simulink model "stateflowrpiv2"  (R2024a)
settings: Solver=FixedStepAuto  StartTime=0.0  StopTime=10.0  RelTol=1e-3  EnableMultiTasking=on
values from neighbouring files (symbols this model uses):
  apps1AdcMax = 30000.0    [rfr25rpi_datadict.sldd]
  apps1AdcMin = 5000.0    [rfr25rpi_datadict.sldd]
  apps2AdcMax = 2000.0    [rfr25rpi_datadict.sldd]
  apps2AdcMin = 1000.0    [rfr25rpi_datadict.sldd]
  cmdTorqueMax = 0.0    [rfr25rpi_datadict.sldd]
  cmdTorqueMin = 5.0    [rfr25rpi_datadict.sldd]
  FDR = 3.77    [rfr25rpi_datadict.sldd]
  MotorRPMtoSpeed = 0.02346    [rfr25rpi_datadict.sldd]
undefined symbols (not defined in the file or in its folder): A0, A2, A3, ended, GND, Single
libraries: raspberrypiBasiclib x9, canmsglib x7, simulink x4, raspberrypiCommlib x3
settings Model: DataDictionary=rfr25rpi_datadict.sldd  ExtModeTrigDuration=2  Creator=user  LastModifiedBy=user
settings SolverCC: PositivePriorityOrder=on
settings OptimizationCC: EnhancedBackFolding=on  PassReuseOutputArgsAs=Individual arguments  ZeroExternalMemoryAtStartup=off  ZeroInternalMemoryAtStartup=off  MaxStackSize=64  OptimizeBlockOrder=speed  DifferentSizesBufferReuse=on  OptimizationCustomize=off  EfficientTunableParamExpr=on
settings DebuggingCC: ParameterTunabilityLossMsg=error
settings HardwareCC: ProdBitPerPointer=32  ProdBitPerSizeT=32  ProdBitPerPtrDiffT=32  ProdLargestAtomicInteger=Long  ProdLargestAtomicFloat=Double  ProdWordSize=32  ProdLongLongMode=on  ProdHWDeviceType=ARM Compatible->ARM Cortex
settings RTWCC: Description=Embedded Coder  SystemTargetFile=ert.tlc  HardwareBoard=Raspberry Pi  TLCOptions="-aInlineSetEventsForThisBaseRateFcn=TLC_FALSE -aSuppressMultiTaskScheduler=TLC_FALSE  -aRateBasedStepFcn=0"  TemplateMakefile=ert_default_tmf  Toolchain=GNU GCC Embedded Linux  BuildConfiguration=Faster Runs
settings CodeAppCC: ForceParamTrailComments=on  IgnoreCustomStorageClasses=off  OperatorAnnotations=on  SimulinkDataObjDesc=on  SFDataObjDesc=on  InsertBlockDesc=on
settings ERTTargetCC: SupportVariableSizeSignals=on

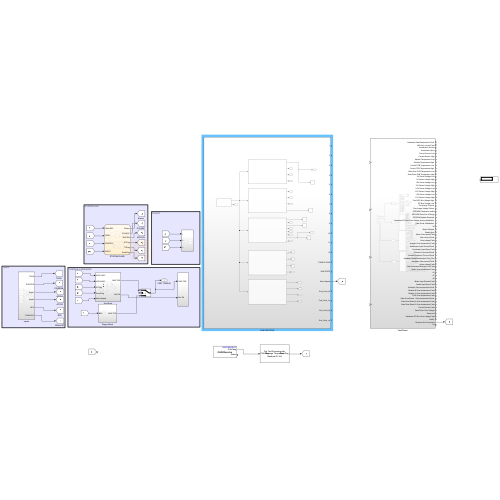
[thumbnail: Simulink's stored preview of the top-level diagram]
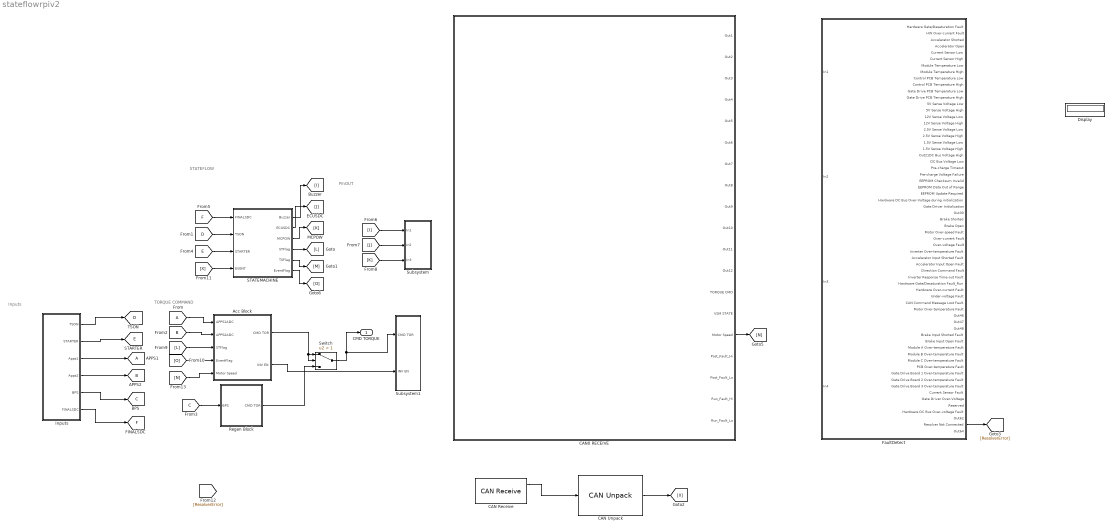
== system stateflowrpiv2 ==
  note: STATEFLOW
  note: TORQUE COMMAND
  note: Inputs
  note: PinOUT
  APPS1 : Goto  TagVisibility=global
  Acc Block : Subsystem
  CAN Receive : raspberrypiCommlib/CAN Receive  DeviceID=can1  SetupCAN=off  TypeofCAN=Real  OutputDataType=CAN Msg  IdentifierType=Standard (11-bit identifier)  MessageId=100  MsgLength=8  SampleTime=-1  OutputError=off  OutputRemote=off  SimulateUsing=Code generation
  CAN Unpack : canmsglib/CAN Unpack  CANdbFile=E:\EE2025\TestTorquemap.dbc  MsgList=TorqueMap  MsgName=TorqueMap  MsgIDType=Standard (11-bit identifier)  MsgIdentifier=244  MsgLength=1  SignalInfo={'EventFlag','0','8','LE','unsigned','Standard','0','1','0','0','255'}  IDPort=off  TimestampPort=off  ErrorPort=off  RemotePort=off  LengthPort=off  StatusPort=off  ApplyMinMax=off
      settings: LibrarySourceBlock=canlib/CAN Unpack  DataFormat=CANdb specified signals
  CAN0 RECEIVE : Subsystem
  Display : Display
  FaultDetect : Subsystem
  From : From  TagVisibility=global
  Inputs : Subsystem
  Regen Block : Subsystem
  STATEMACHINE : Stateflow chart  TreatAsAtomicUnit=on
      settings: PortSchema="{\"entries\":[{\"content\":{\"sides\":[{\"content\":{\"connectorIds\":[\"In1\",\"In2\",\"In3\",\"In4\"]},\"type\":\"ConnectorPlacement.EquallySpacedRectSide\",\"uuid\":\"0f8b280b-7cb1-472e-a5ac-e36a5d7bcf1b\"},{\"content\":{\"connectorIds\":[\"Out1\",\"Out5\",\"Out3\",\"Out4\",\"Out2\",\"Out6\"],\"side\":\"RIGHT\"},\"type\":\"ConnectorPlacement.EquallySpacedRectSide\",\"uuid\":\"0b1c52b6-a8da-4f2c-8787-2a587349ccd1\"},{\"content\":{\"side\":\"TOP\"},\"type\":\"ConnectorPlacement.EquallySpacedRectSide\",\"uuid\":\"6fa40707-83f4-478b-9f22-811819b1809f\"}]},\"type\":\"ConnectorPlacement.EquallySpacedConnector\",\"uuid\":\"b2952a38-a560-4999-b9e3-ff289dd499fe\"}],\"packageUris\":[\"http://schema.mathworks.com/mf0/Connector/R2020b\"],\"version\":\"1.0\"}"
  Subsystem : Subsystem
  Subsystem1 : Subsystem
  Switch : Switch  Criteria=u2 > Threshold  Threshold=1  SaturateOnIntegerOverflow=off  InputSameDT=off
  CMD TORQUE : Outport
  tag scope: B=global, C=global, D=global, E=global, F=global
  wires:
  [L] -> Acc Block/3(STFlag)
  [E] -> STATEMACHINE/3(STARTER)
  Regen Block/1(CMD TOR) -> Switch/3
  STATEMACHINE/2(TSFlag) -> [M]
  Acc Block/2(INV EN) -> Subsystem1/2(INV EN)
  Inputs/2(STARTER) -> [E]
  STATEMACHINE/5(ECUSDC) -> [J]
  STATEMACHINE/1(Buzzer) -> [I]
  Inputs/6(FINALSDC) -> [F]
  [J] -> Subsystem/2(In2)
  [D] -> STATEMACHINE/2(TSON)
  Inputs/3(Apps1) -> APPS1/1
  Inputs/1(TSON) -> [D]
  [C] -> Regen Block/1(BPS)
  STATEMACHINE/3(MCPOW) -> [K]
  [I] -> Subsystem/1(In1)
  Inputs/4(Apps2) -> [B]
  [F] -> STATEMACHINE/1(FINALSDC)
  [B] -> Acc Block/2(APPS2ADC)
  Inputs/5(BPS) -> [C]
  [K] -> Subsystem/3(In3)
  Acc Block/1(CMD TOR) -> Switch/2, Switch/1
  STATEMACHINE/4(STFlag) -> [L]
  From/1 -> Acc Block/1(APPS1ADC)
  Switch/1 -> CMD TORQUE/1, Subsystem1/1(CMD TOR)
  [N] -> Acc Block/5(Motor Speed)
  STATEMACHINE/6(EventFlag) -> [O]
  [O] -> Acc Block/4(EventFlag)
  CAN0 RECEIVE/15(Motor Speed) -> [N]
  CAN Receive/1 -> CAN Unpack/1
  CAN Unpack/1 -> [X]
  [X] -> STATEMACHINE/4(EVENT)
  FaultDetect/63(Resolver Not Connected) -> [ResolverError]

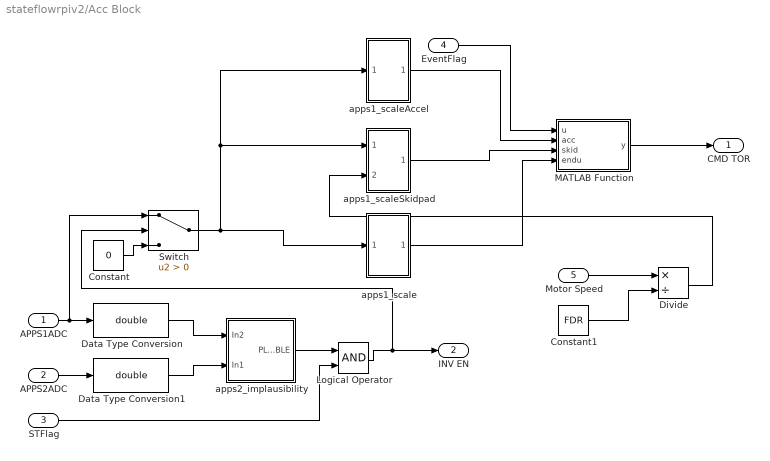
== system stateflowrpiv2/Acc Block ==
  APPS1ADC : Inport
  APPS2ADC : Inport  Port=2
  STFlag : Inport  Port=3
  EventFlag : Inport  Port=4
  Motor Speed : Inport  Port=5
  Constant : Constant  Value=0
  Constant1 : Constant  Value=FDR
  Data Type Conversion : DataTypeConversion  OutDataTypeStr=double  SaturateOnIntegerOverflow=off  RndMeth=Floor
  Data Type Conversion1 : DataTypeConversion  OutDataTypeStr=double  SaturateOnIntegerOverflow=off  RndMeth=Floor
  Divide : Product  Inputs=*/
  Logical Operator : Logic  AllPortsSameDT=off  OutDataTypeStr=boolean
  MATLAB Function : MATLAB Function  TreatAsAtomicUnit=on
  Switch : Switch  Criteria=u2 > Threshold  SaturateOnIntegerOverflow=off  InputSameDT=off
  apps1_scale : Subsystem
  apps1_scaleAccel : Subsystem
  apps1_scaleSkidpad : Subsystem
  apps2_implausibility : Subsystem
  CMD TOR : Outport
  INV EN : Outport  Port=2
  wires:
  APPS1ADC/1 -> Switch/1, Data Type Conversion/1
  APPS2ADC/1 -> Data Type Conversion1/1
  Data Type Conversion1/1 -> apps2_implausibility/2(In1)
  Data Type Conversion/1 -> apps2_implausibility/1(In2)
  apps2_implausibility/1(PLAUSIBLE) -> Logical Operator/1
  Constant/1 -> Switch/3
  STFlag/1 -> Logical Operator/2
  Logical Operator/1 -> Switch/2, INV EN/1
  Motor Speed/1 -> Divide/1
  Constant1/1 -> Divide/2
  Divide/1 -> apps1_scaleSkidpad/2(In2)
  Switch/1 -> apps1_scale/1(In1), apps1_scaleSkidpad/1(In1), apps1_scaleAccel/1(In1)
  EventFlag/1 -> MATLAB Function/1(u)
  apps1_scaleAccel/1(acc) -> MATLAB Function/2(acc)
  apps1_scaleSkidpad/1(skid) -> MATLAB Function/3(skid)
  apps1_scale/1(endu) -> MATLAB Function/4(endu)
  MATLAB Function/1(y) -> CMD TOR/1

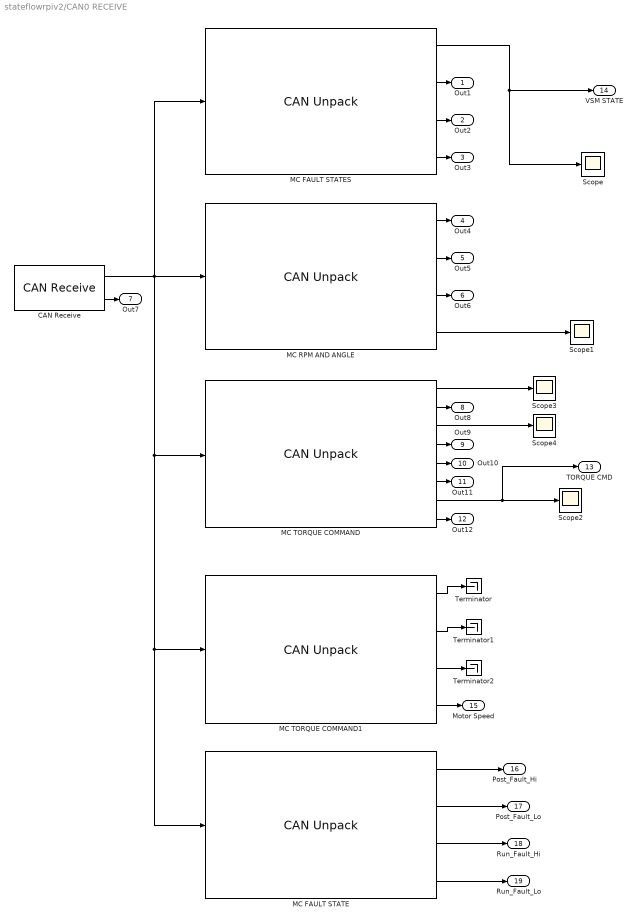
== system stateflowrpiv2/CAN0 RECEIVE ==
  CAN Receive : raspberrypiCommlib/CAN Receive  DeviceID=can0  SetupCAN=on  TypeofCAN=Real  OutputDataType=CAN Msg  IdentifierType=Standard (11-bit identifier)  MessageId=100  MsgLength=8  SampleTime=-1  OutputError=off  OutputRemote=off  SimulateUsing=Code generation
  MC FAULT STATE : canmsglib/CAN Unpack  CANdbFile=C:\Users\user\Desktop\rfr25can0.dbc  MsgList=M171_Fault_Codes  MsgName=M171_Fault_Codes  MsgIDType=Standard (11-bit identifier)  MsgIdentifier=171  MsgLength=8  SignalInfo={'INV_Post_Fault_Hi','16','16','LE','unsigned','Standard','0','1','0','0','65535';'INV_Post_Fault_Lo','0','16','LE','unsigned','Standard','0','1','0','0','65535';'INV_Run_Fault_Hi','48','16','LE','unsigned','Standard','0','1','0','0','65535';'INV_Run_Fault_Lo','32','16','LE','unsigned','Standard','0','1','0','0','65535'}  IDPort=off  TimestampPort=off  ErrorPort=off  RemotePort=off  LengthPort=off  StatusPort=off  ApplyMinMax=off
      settings: LibrarySourceBlock=canlib/CAN Unpack  DataFormat=CANdb specified signals
  MC FAULT STATES : canmsglib/CAN Unpack  CANdbFile=C:\Users\1724a\OneDrive\Desktop\rfr\rfr25can0.dbc  MsgList=(none)  MsgName=M171_Fault_Codes  MsgIDType=Standard (11-bit identifier)  MsgIdentifier=171  MsgLength=8  SignalInfo={'INV_Post_Fault_Hi','16','16','LE','unsigned','Standard','0','1','0','0','65535';'INV_Post_Fault_Lo','0','16','LE','unsigned','Standard','0','1','0','0','65535';'INV_Run_Fault_Hi','48','16','LE','unsigned','Standard','0','1','0','0','65535';'INV_Run_Fault_Lo','32','16','LE','unsigned','Standard','0','1','0','0','65535'}  IDPort=off  TimestampPort=off  ErrorPort=off  RemotePort=off  LengthPort=off  StatusPort=off  ApplyMinMax=off
      settings: LibrarySourceBlock=canlib/CAN Unpack  DataFormat=CANdb specified signals
  MC RPM AND ANGLE : canmsglib/CAN Unpack  CANdbFile=C:\Users\1724a\OneDrive\Desktop\rfr\rfr25can0.dbc  MsgList=(none)  MsgName=M165_Motor_Position_Info  MsgIDType=Standard (11-bit identifier)  MsgIdentifier=165  MsgLength=8  SignalInfo={'INV_Delta_Resolver_Filtered','48','16','LE','signed','Standard','0','0.1','0','-3276.8','3276.7';'INV_Electrical_Output_Frequency','32','16','LE','signed','Standard','0','0.1','0','-3276.8','3276.7';'INV_Motor_Angle_Electrical','0','16','LE','unsigned','Standard','0','0.1','0','0','6553.5';'INV_Motor_Speed','16','16','LE','signed','Standard','0','1','0','-32768','32767'}  IDPort=off  TimestampPort=off  ErrorPort=off  RemotePort=off  LengthPort=off  StatusPort=off  ApplyMinMax=off
      settings: LibrarySourceBlock=canlib/CAN Unpack  DataFormat=CANdb specified signals
  MC TORQUE COMMAND : canmsglib/CAN Unpack  CANdbFile=C:\Users\1724a\OneDrive\Desktop\rfr\rfr25can0.dbc  MsgList=(none)  MsgName=M192_Command_Message  MsgIDType=Standard (11-bit identifier)  MsgIdentifier=192  MsgLength=8  SignalInfo={'VCU_INV_Direction_Command','32','1','LE','unsigned','Standard','0','1','0','0','1';'VCU_INV_Inverter_Discharge','41','1','LE','unsigned','Standard','0','1','0','0','1';'VCU_INV_Inverter_Enable','40','1','LE','unsigned','Standard','0','1','0','0','1';'VCU_INV_RollingCounter','44','4','LE','unsigned','Standard','0','1','0','0','15';'VCU_INV_Speed_Command','16','16','LE','signed','Standard','0','1','0','-32768','32767';'VCU_INV_Speed_Mode_Enable','42','1','LE','unsigned','Standard','0','1','0','0','1';'VCU_INV_Torque_Command','0','16','LE','signed','Standard','0','0.1','0','-3276.8','3276.7';'VCU_INV_Torque_Limit_Command','48','16','LE','signed','Standard','0','0.1','0','-3276.8','3276.7'}  IDPort=off  TimestampPort=off  ErrorPort=off  RemotePort=off  LengthPort=off  StatusPort=off  ApplyMinMax=off
      settings: LibrarySourceBlock=canlib/CAN Unpack  DataFormat=CANdb specified signals
  MC TORQUE COMMAND1 : canmsglib/CAN Unpack  CANdbFile=C:\Users\user\Desktop\rfr25can0.dbc  MsgList=M165_Motor_Position_Info  MsgName=M165_Motor_Position_Info  MsgIDType=Standard (11-bit identifier)  MsgIdentifier=165  MsgLength=8  SignalInfo={'INV_Delta_Resolver_Filtered','48','16','LE','signed','Standard','0','0.1','0','-3276.8','3276.7';'INV_Electrical_Output_Frequency','32','16','LE','signed','Standard','0','0.1','0','-3276.8','3276.7';'INV_Motor_Angle_Electrical','0','16','LE','unsigned','Standard','0','0.1','0','0','6553.5';'INV_Motor_Speed','16','16','LE','signed','Standard','0','1','0','-32768','32767'}  IDPort=off  TimestampPort=off  ErrorPort=off  RemotePort=off  LengthPort=off  StatusPort=off  ApplyMinMax=off
      settings: LibrarySourceBlock=canlib/CAN Unpack  DataFormat=CANdb specified signals
  Scope{,1..4} (5 alike) : Scope
  Terminator : Terminator
  Terminator1 : Terminator
  Terminator2 : Terminator
  Out1 : Outport
  Out2 : Outport  Port=2
  Out3 : Outport  Port=3
  Out4 : Outport  Port=4
  Out5 : Outport  Port=5
  Out6 : Outport  Port=6
  Out7 : Outport  Port=7
  Out8 : Outport  Port=8
  Out9 : Outport  Port=9
  Out10 : Outport  Port=10
  Out11 : Outport  Port=11
  Out12 : Outport  Port=12
  TORQUE CMD : Outport  Port=13
  VSM STATE : Outport  Port=14
  Motor Speed : Outport  Port=15
  Post_Fault_Hi : Outport  Port=16
  Post_Fault_Lo : Outport  Port=17
  Run_Fault_Hi : Outport  Port=18
  Run_Fault_Lo : Outport  Port=19
  wires:
  MC TORQUE COMMAND/3 -> Scope4/1
  CAN Receive/1 -> MC TORQUE COMMAND1/1, MC FAULT STATE/1, MC TORQUE COMMAND/1, MC FAULT STATES/1, MC RPM AND ANGLE/1
  MC TORQUE COMMAND/8 -> Out12/1
  MC TORQUE COMMAND/4 -> Out9/1
  MC RPM AND ANGLE/2 -> Out5/1
  MC TORQUE COMMAND/1 -> Scope3/1
  MC RPM AND ANGLE/1 -> Out4/1
  MC FAULT STATES/1 -> VSM STATE/1, Scope/1
  MC TORQUE COMMAND/6 -> Out11/1
  MC RPM AND ANGLE/4 -> Scope1/1
  MC FAULT STATES/3 -> Out2/1
  CAN Receive/2 -> Out7/1
  MC FAULT STATES/2 -> Out1/1
  MC TORQUE COMMAND/2 -> Out8/1
  MC FAULT STATES/4 -> Out3/1
  MC TORQUE COMMAND/5 -> Out10/1
  MC RPM AND ANGLE/3 -> Out6/1
  MC TORQUE COMMAND/7 -> TORQUE CMD/1, Scope2/1
  MC TORQUE COMMAND1/4 -> Motor Speed/1
  MC TORQUE COMMAND1/1 -> Terminator/1
  MC TORQUE COMMAND1/2 -> Terminator1/1
  MC TORQUE COMMAND1/3 -> Terminator2/1
  MC FAULT STATE/2 -> Post_Fault_Lo/1
  MC FAULT STATE/3 -> Run_Fault_Hi/1
  MC FAULT STATE/4 -> Run_Fault_Lo/1
  MC FAULT STATE/1 -> Post_Fault_Hi/1

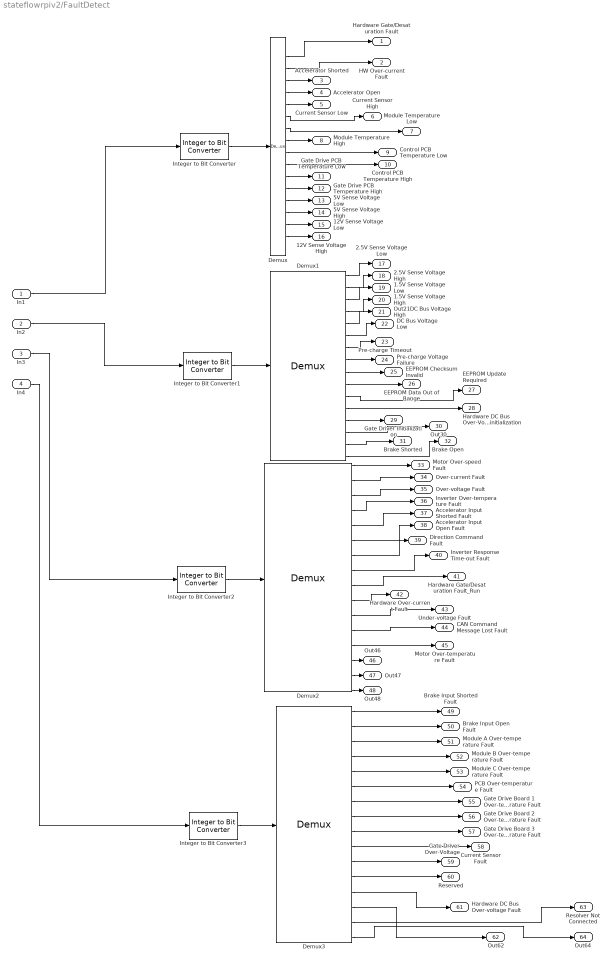
== system stateflowrpiv2/FaultDetect ==
  In1 : Inport
  In2 : Inport  Port=2
  In3 : Inport  Port=3
  In4 : Inport  Port=4
  Demux{,1..3} (4 alike) : Demux  Outputs=16
  Integer to Bit Converter{,1..3} (4 alike) : simulink/Logic and Bit Operations/Integer to Bit Converter  nbits=16  signedInputValues=Unsigned  bitOrder=MSB first  outDtype=Inherit via internal rule
  "Hardware Gate/Desaturation Fault " : Outport
  HW Over-current Fault : Outport  Port=2
  Accelerator Shorted : Outport  Port=3
  Accelerator Open : Outport  Port=4
  Current Sensor Low : Outport  Port=5
  Current Sensor High : Outport  Port=6
  Module Temperature Low : Outport  Port=7
  "Module Temperature High " : Outport  Port=8
  "Control PCB Temperature Low " : Outport  Port=9
  "Control PCB Temperature High " : Outport  Port=10
  Gate Drive PCB Temperature Low : Outport  Port=11
  Gate Drive PCB Temperature High : Outport  Port=12
  5V Sense Voltage Low : Outport  Port=13
  5V Sense Voltage High : Outport  Port=14
  12V Sense Voltage Low : Outport  Port=15
  12V Sense Voltage High : Outport  Port=16
  2.5V Sense Voltage Low : Outport  Port=17
  2.5V Sense Voltage High : Outport  Port=18
  1.5V Sense Voltage Low : Outport  Port=19
  1.5V Sense Voltage High : Outport  Port=20
  "Out21DC Bus Voltage High " : Outport  Port=21
  "DC Bus Voltage Low " : Outport  Port=22
  "Pre-charge Timeout " : Outport  Port=23
  "Pre-charge Voltage Failure " : Outport  Port=24
  EEPROM Checksum Invalid : Outport  Port=25
  EEPROM Data Out of Range : Outport  Port=26
  "EEPROM Update Required " : Outport  Port=27
  "Hardware DC Bus Over-Voltage during initialization " : Outport  Port=28
  "Gate Driver Initialization " : Outport  Port=29
  Out30 : Outport  Port=30
  "Brake Shorted " : Outport  Port=31
  Brake Open : Outport  Port=32
  Motor Over-speed Fault : Outport  Port=33
  "Over-current Fault " : Outport  Port=34
  Over-voltage Fault : Outport  Port=35
  Inverter Over-temperature Fault : Outport  Port=36
  "Accelerator Input Shorted Fault " : Outport  Port=37
  Accelerator Input Open Fault : Outport  Port=38
  "Direction Command Fault " : Outport  Port=39
  "Inverter Response Time-out Fault " : Outport  Port=40
  Hardware Gate/Desaturation Fault_Run : Outport  Port=41
  "Hardware Over-current Fault " : Outport  Port=42
  Under-voltage Fault : Outport  Port=43
  CAN Command Message Lost Fault : Outport  Port=44
  Motor Over-temperature Fault : Outport  Port=45
  Out46 : Outport  Port=46
  Out47 : Outport  Port=47
  Out48 : Outport  Port=48
  Brake Input Shorted Fault : Outport  Port=49
  Brake Input Open Fault : Outport  Port=50
  "Module A Over-temperature Fault " : Outport  Port=51
  Module B Over-temperature Fault : Outport  Port=52
  Module C Over-temperature Fault : Outport  Port=53
  PCB Over-temperature Fault : Outport  Port=54
  "Gate Drive Board 1 Over-temperature Fault " : Outport  Port=55
  Gate Drive Board 2 Over-temperature Fault : Outport  Port=56
  Gate Drive Board 3 Over-temperature Fault : Outport  Port=57
  Current Sensor Fault : Outport  Port=58
  Gate Driver Over-Voltage : Outport  Port=59
  Reserved : Outport  Port=60
  Hardware DC Bus Over-voltage Fault : Outport  Port=61
  "Out62 " : Outport  Port=62
  Resolver Not Connected : Outport  Port=63
  Out64 : Outport  Port=64
  wires:
  Demux2/7 -> "Direction Command Fault "/1
  Demux3/9 -> Gate Drive Board 3 Over-temperature Fault/1
  Integer to Bit Converter1/1 -> Demux1/1
  Demux/4 -> Accelerator Open/1
  Demux/2 -> HW Over-current Fault/1
  Demux1/14 -> Out30/1
  Demux/13 -> 5V Sense Voltage Low/1
  Demux/9 -> "Control PCB Temperature Low "/1
  Demux2/1 -> Motor Over-speed Fault/1
  Demux3/2 -> Brake Input Open Fault/1
  Demux/3 -> Accelerator Shorted/1
  Integer to Bit Converter/1 -> Demux/1
  Demux3/13 -> Hardware DC Bus Over-voltage Fault/1
  Demux1/15 -> "Brake Shorted "/1
  Demux1/9 -> EEPROM Checksum Invalid/1
  Demux1/12 -> "Hardware DC Bus Over-Voltage during initialization "/1
  Demux/5 -> Current Sensor Low/1
  Demux2/10 -> "Hardware Over-current Fault "/1
  Demux/15 -> 12V Sense Voltage Low/1
  Demux/6 -> Current Sensor High/1
  Integer to Bit Converter2/1 -> Demux2/1
  Demux2/13 -> Motor Over-temperature Fault/1
  Integer to Bit Converter3/1 -> Demux3/1
  Demux/16 -> 12V Sense Voltage High/1
  In1/1 -> Integer to Bit Converter/1
  Demux/14 -> 5V Sense Voltage High/1
  Demux1/3 -> 1.5V Sense Voltage Low/1
  Demux3/7 -> "Gate Drive Board 1 Over-temperature Fault "/1
  Demux1/1 -> 2.5V Sense Voltage Low/1
  Demux3/8 -> Gate Drive Board 2 Over-temperature Fault/1
  Demux2/5 -> "Accelerator Input Shorted Fault "/1
  Demux1/6 -> "DC Bus Voltage Low "/1
  Demux2/8 -> "Inverter Response Time-out Fault "/1
  Demux3/5 -> Module C Over-temperature Fault/1
  Demux/11 -> Gate Drive PCB Temperature Low/1
  Demux/8 -> "Module Temperature High "/1
  Demux3/12 -> Reserved/1
  Demux3/1 -> Brake Input Shorted Fault/1
  Demux1/16 -> Brake Open/1
  Demux1/13 -> "Gate Driver Initialization "/1
  Demux/7 -> Module Temperature Low/1
  Demux/1 -> "Hardware Gate/Desaturation Fault "/1
  Demux2/6 -> Accelerator Input Open Fault/1
  Demux2/2 -> "Over-current Fault "/1
  Demux3/4 -> Module B Over-temperature Fault/1
  Demux1/5 -> "Out21DC Bus Voltage High "/1
  Demux2/14 -> Out46/1
  Demux3/3 -> "Module A Over-temperature Fault "/1
  Demux/12 -> Gate Drive PCB Temperature High/1
  Demux1/10 -> EEPROM Data Out of Range/1
  Demux1/8 -> "Pre-charge Voltage Failure "/1
  Demux2/3 -> Over-voltage Fault/1
  Demux2/4 -> Inverter Over-temperature Fault/1
  Demux2/9 -> Hardware Gate/Desaturation Fault_Run/1
  Demux3/6 -> PCB Over-temperature Fault/1
  In2/1 -> Integer to Bit Converter1/1
  Demux3/14 -> "Out62 "/1
  Demux1/11 -> "EEPROM Update Required "/1
  Demux1/7 -> "Pre-charge Timeout "/1
  Demux1/4 -> 1.5V Sense Voltage High/1
  In4/1 -> Integer to Bit Converter3/1
  Demux3/16 -> Out64/1
  Demux3/11 -> Gate Driver Over-Voltage/1
  Demux3/10 -> Current Sensor Fault/1
  Demux/10 -> "Control PCB Temperature High "/1
  Demux2/15 -> Out47/1
  Demux1/2 -> 2.5V Sense Voltage High/1
  Demux2/11 -> Under-voltage Fault/1
  Demux2/12 -> CAN Command Message Lost Fault/1
  Demux2/16 -> Out48/1
  Demux3/15 -> Resolver Not Connected/1
  In3/1 -> Integer to Bit Converter2/1

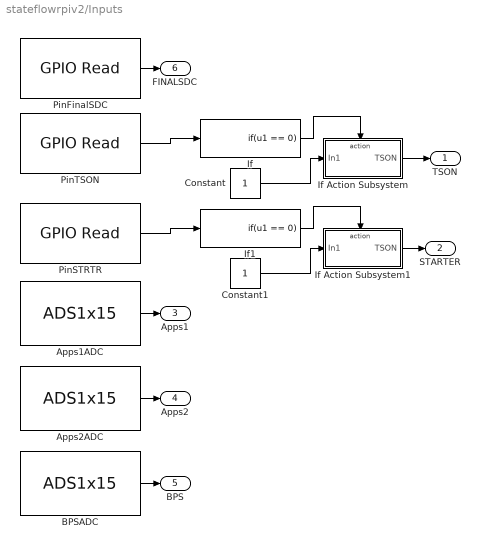
== system stateflowrpiv2/Inputs ==
  Apps1ADC : raspberrypiBasiclib/ADS1x15  ADCChip=ADS1115  I2CAddress=0x48  ConversionMode=Single-shot  InputConfiguration=A2 - GND (Single-ended)  GainConfigurationDifferential=+/- 2.048 V  GainConfigurationSingleEnded=1.024 V  DataRateConfigurationADS1015=1600SPS  DataRateConfigurationADS1115=860SPS  SampleTime=0.1  EnableComparatorMode=off  ComparatorMode=Traditional with hysterisis  ComparatorPolarityConfiguration=Active low  ComparatorLatchingConfiguration=Non-latching  ComparatorQueueConfiguration=Assert after 1 conversion  ComparatorLowThresholdADS1015=0  ComparatorLowThresholdADS1115=0  ComparatorHighThresholdADS1015=0  ComparatorHighThresholdADS1115=0
  Apps2ADC : raspberrypiBasiclib/ADS1x15  ADCChip=ADS1115  I2CAddress=0x48  ConversionMode=Single-shot  InputConfiguration=A3 - GND (Single-ended)  GainConfigurationDifferential=+/- 2.048 V  GainConfigurationSingleEnded=1.024 V  DataRateConfigurationADS1015=1600SPS  DataRateConfigurationADS1115=860SPS  SampleTime=0.1  EnableComparatorMode=off  ComparatorMode=Traditional with hysterisis  ComparatorPolarityConfiguration=Active low  ComparatorLatchingConfiguration=Non-latching  ComparatorQueueConfiguration=Assert after 1 conversion  ComparatorLowThresholdADS1015=0  ComparatorLowThresholdADS1115=0  ComparatorHighThresholdADS1015=0  ComparatorHighThresholdADS1115=0
  BPSADC : raspberrypiBasiclib/ADS1x15  ADCChip=ADS1115  I2CAddress=0x48  ConversionMode=Single-shot  InputConfiguration=A0 - GND (Single-ended)  GainConfigurationDifferential=+/- 2.048 V  GainConfigurationSingleEnded=1.024 V  DataRateConfigurationADS1015=1600SPS  DataRateConfigurationADS1115=860SPS  SampleTime=0.1  EnableComparatorMode=off  ComparatorMode=Traditional with hysterisis  ComparatorPolarityConfiguration=Active low  ComparatorLatchingConfiguration=Non-latching  ComparatorQueueConfiguration=Assert after 1 conversion  ComparatorLowThresholdADS1015=0  ComparatorLowThresholdADS1115=0  ComparatorHighThresholdADS1015=0  ComparatorHighThresholdADS1115=0
  Constant : Constant
  Constant1 : Constant
  If : If  IfExpression=u1 == 0  ShowElse=off
  If Action Subsystem : Subsystem  TreatAsAtomicUnit=on
  If Action Subsystem1 : Subsystem  TreatAsAtomicUnit=on
  If1 : If  IfExpression=u1 == 0  ShowElse=off
  PinFinalSDC : raspberrypiBasiclib/GPIO Read  board=Pi Zero 2 W  gpio=5  internalResistor=Off  sampleTime=0.1  direction=Input  blockPlatform=Raspberry Pi
  PinSTRTR : raspberrypiBasiclib/GPIO Read  board=Pi Zero 2 W  gpio=12  internalResistor=Off  sampleTime=0.1  direction=Input  blockPlatform=Raspberry Pi
  PinTSON : raspberrypiBasiclib/GPIO Read  board=Pi Zero 2 W  gpio=13  internalResistor=Off  sampleTime=0.1  direction=Input  blockPlatform=Raspberry Pi
  TSON : Outport
  STARTER : Outport  Port=2
  Apps1 : Outport  Port=3
  Apps2 : Outport  Port=4
  BPS : Outport  Port=5
  FINALSDC : Outport  Port=6
  wires:
  Apps2ADC/1 -> Apps2/1
  Apps1ADC/1 -> Apps1/1
  BPSADC/1 -> BPS/1
  PinFinalSDC/1 -> FINALSDC/1
  PinTSON/1 -> If/1
  If/1 -> If Action Subsystem/Action
  Constant/1 -> If Action Subsystem/1(In1)
  If Action Subsystem/1(TSON) -> TSON/1
  PinSTRTR/1 -> If1/1
  If Action Subsystem1/1(TSON) -> STARTER/1
  Constant1/1 -> If Action Subsystem1/1(In1)
  If1/1 -> If Action Subsystem1/Action

== system stateflowrpiv2/Regen Block ==
  BPS : Inport
  Data Type Conversion : DataTypeConversion  OutDataTypeStr=double  SaturateOnIntegerOverflow=off  RndMeth=Floor
  Scope : Scope
  Scope1 : Scope
  apps_scale : Subsystem
  CMD TOR : Outport
  wires:
  Data Type Conversion/1 -> apps_scale/1(In1), Scope/1
  apps_scale/1(Out1) -> CMD TOR/1, Scope1/1
  BPS/1 -> Data Type Conversion/1

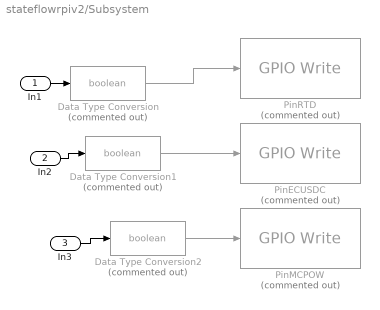
== system stateflowrpiv2/Subsystem ==
  In1 : Inport
  In2 : Inport  Port=2
  In3 : Inport  Port=3
  Data Type Conversion : DataTypeConversion  Commented=on  OutDataTypeStr=boolean  SaturateOnIntegerOverflow=off  RndMeth=Floor
  Data Type Conversion1 : DataTypeConversion  Commented=on  OutDataTypeStr=boolean  SaturateOnIntegerOverflow=off  RndMeth=Floor
  Data Type Conversion2 : DataTypeConversion  Commented=on  OutDataTypeStr=boolean  SaturateOnIntegerOverflow=off  RndMeth=Floor
  PinECUSDC : raspberrypiBasiclib/GPIO Write  Commented=on  board=Pi Zero 2 W  gpio=17  direction=Output  blockPlatform=Raspberry Pi
  PinMCPOW : raspberrypiBasiclib/GPIO Write  Commented=on  board=Pi Zero 2 W  gpio=6  direction=Output  blockPlatform=Raspberry Pi
  PinRTD : raspberrypiBasiclib/GPIO Write  Commented=on  board=Pi Zero 2 W  gpio=25  direction=Output  blockPlatform=Raspberry Pi
  wires:
  In1/1 -> Data Type Conversion/1
  Data Type Conversion/1 -> PinRTD/1
  Data Type Conversion1/1 -> PinECUSDC/1
  In2/1 -> Data Type Conversion1/1
  Data Type Conversion2/1 -> PinMCPOW/1
  In3/1 -> Data Type Conversion2/1

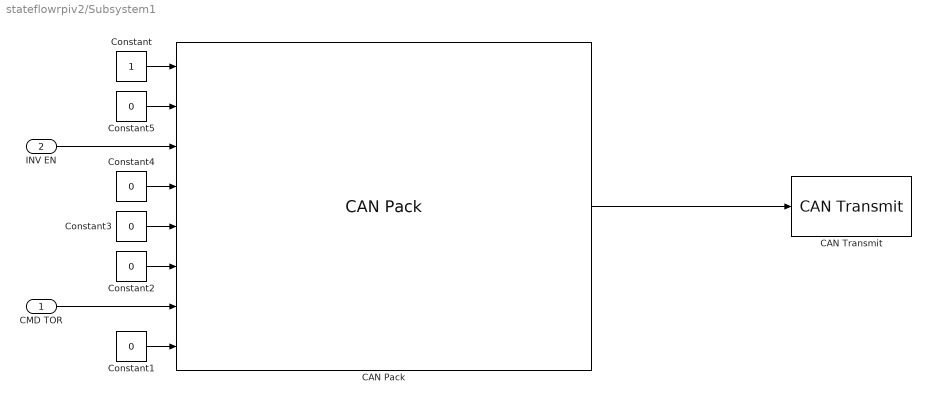
== system stateflowrpiv2/Subsystem1 ==
  CMD TOR : Inport
  INV EN : Inport  Port=2
  CAN Pack : canmsglib/CAN Pack  CANdbFile=C:\Users\user\Desktop\rfr25can0.dbc  MsgList=(none)  MsgName=M192_Command_Message  MsgIDType=Standard (11-bit identifier)  MsgIdentifier=192  MsgLength=8  Remote=off  ApplyMinMax=off  BusOutput=on  SignalInfo={'VCU_INV_Direction_Command','32','1','LE','unsigned','Standard','0','1','0','0','1';'VCU_INV_Inverter_Discharge','41','1','LE','unsigned','Standard','0','1','0','0','1';'VCU_INV_Inverter_Enable','40','1','LE','unsigned','Standard','0','1','0','0','1';'VCU_INV_RollingCounter','44','4','LE','unsigned','Standard','0','1','0','0','15';'VCU_INV_Speed_Command','16','16','LE','signed','Standard','0','1','0','-32768','32767';'VCU_INV_Speed_Mode_Enable','42','1','LE','unsigned','Standard','0','1','0','0','1';'VCU_INV_Torque_Command','0','16','LE','signed','Standard','0','0.1','0','-3276.8','3276.7';'VCU_INV_Torque_Limit_Command','48','16','LE','signed','Standard','0','0.1','0','-3276.8','3276.7'}
      settings: LibrarySourceBlock=canlib/CAN Pack  DataFormat=CANdb specified signals
  CAN Transmit : raspberrypiCommlib/CAN Transmit  DeviceID=can0  SetupCAN=on  TypeofCAN=Real  InputDataType=CAN Msg  BlockingMode_=on  BlockTimeout_=100  OutputStatus=off  IdentifierType=Standard (11-bit identifier)  MessageId=192  MsgLength=8  RemoteFrame=off  SimulateUsing=Code generation
  Constant : Constant
  Constant{1..5} (5 alike) : Constant  Value=0
  wires:
  ? -> ?
  Constant5/1 -> CAN Pack/2
  Constant3/1 -> CAN Pack/5
  Constant4/1 -> CAN Pack/4
  Constant1/1 -> CAN Pack/8
  CMD TOR/1 -> CAN Pack/7
  INV EN/1 -> CAN Pack/3
  Constant/1 -> CAN Pack/1
  Constant2/1 -> CAN Pack/6
  CAN Pack/1 -> CAN Transmit/1

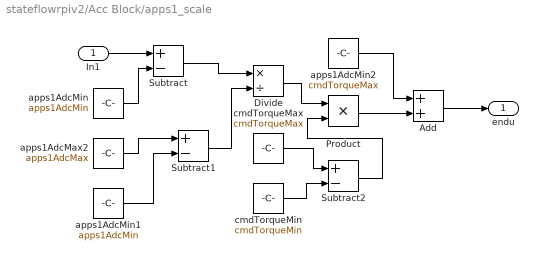
== system stateflowrpiv2/Acc Block/apps1_scale ==
  In1 : Inport
  Add : Sum
  Divide : Product  Inputs=*/
  Product : Product
  Subtract : Sum  Inputs=+-
  Subtract1 : Sum  Inputs=+-
  Subtract2 : Sum  Inputs=+-
  apps1AdcMax2 : Constant  Value=apps1AdcMax
  apps1AdcMin : Constant  Value=apps1AdcMin
  apps1AdcMin1 : Constant  Value=apps1AdcMin
  apps1AdcMin2 : Constant  Value=cmdTorqueMax
  cmdTorqueMax : Constant  Value=cmdTorqueMax
  cmdTorqueMin : Constant  Value=cmdTorqueMin
  endu : Outport
  wires:
  Add/1 -> endu/1
  Product/1 -> Add/2
  apps1AdcMin1/1 -> Subtract1/2
  apps1AdcMin/1 -> Subtract/2
  Subtract1/1 -> Divide/2
  Divide/1 -> Product/1
  apps1AdcMax2/1 -> Subtract1/1
  cmdTorqueMin/1 -> Subtract2/2
  Subtract2/1 -> Product/2
  cmdTorqueMax/1 -> Subtract2/1
  Subtract/1 -> Divide/1
  apps1AdcMin2/1 -> Add/1
  In1/1 -> Subtract/1

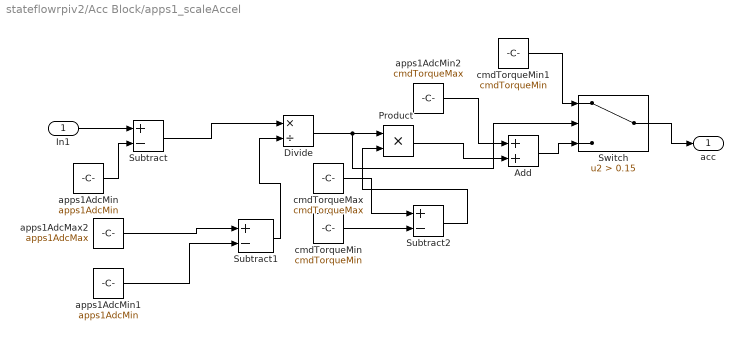
== system stateflowrpiv2/Acc Block/apps1_scaleAccel ==
  In1 : Inport
  Add : Sum
  Divide : Product  Inputs=*/
  Product : Product
  Subtract : Sum  Inputs=+-
  Subtract1 : Sum  Inputs=+-
  Subtract2 : Sum  Inputs=+-
  Switch : Switch  Criteria=u2 > Threshold  Threshold=0.15  SaturateOnIntegerOverflow=off  InputSameDT=off
  apps1AdcMax2 : Constant  Value=apps1AdcMax
  apps1AdcMin : Constant  Value=apps1AdcMin
  apps1AdcMin1 : Constant  Value=apps1AdcMin
  apps1AdcMin2 : Constant  Value=cmdTorqueMax
  cmdTorqueMax : Constant  Value=cmdTorqueMax
  cmdTorqueMin : Constant  Value=cmdTorqueMin
  cmdTorqueMin1 : Constant  Value=cmdTorqueMin
  acc : Outport
  wires:
  Product/1 -> Add/2
  apps1AdcMin1/1 -> Subtract1/2
  apps1AdcMin/1 -> Subtract/2
  Subtract1/1 -> Divide/2
  apps1AdcMax2/1 -> Subtract1/1
  cmdTorqueMin/1 -> Subtract2/2
  Subtract2/1 -> Product/2
  cmdTorqueMax/1 -> Subtract2/1
  Subtract/1 -> Divide/1
  apps1AdcMin2/1 -> Add/1
  In1/1 -> Subtract/1
  Divide/1 -> Switch/2, Product/1
  Add/1 -> Switch/3
  cmdTorqueMin1/1 -> Switch/1
  Switch/1 -> acc/1

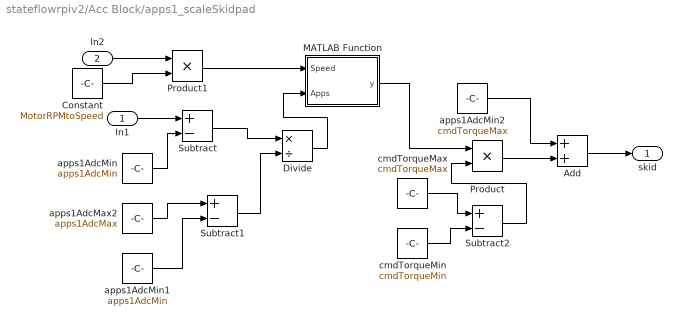
== system stateflowrpiv2/Acc Block/apps1_scaleSkidpad ==
  In1 : Inport
  In2 : Inport  Port=2
  Add : Sum
  Constant : Constant  Value=MotorRPMtoSpeed
  Divide : Product  Inputs=*/
  MATLAB Function : MATLAB Function  TreatAsAtomicUnit=on
  Product : Product
  Product1 : Product
  Subtract : Sum  Inputs=+-
  Subtract1 : Sum  Inputs=+-
  Subtract2 : Sum  Inputs=+-
  apps1AdcMax2 : Constant  Value=apps1AdcMax
  apps1AdcMin : Constant  Value=apps1AdcMin
  apps1AdcMin1 : Constant  Value=apps1AdcMin
  apps1AdcMin2 : Constant  Value=cmdTorqueMax
  cmdTorqueMax : Constant  Value=cmdTorqueMax
  cmdTorqueMin : Constant  Value=cmdTorqueMin
  skid : Outport
  wires:
  Add/1 -> skid/1
  Product/1 -> Add/2
  apps1AdcMin1/1 -> Subtract1/2
  apps1AdcMin/1 -> Subtract/2
  Subtract1/1 -> Divide/2
  apps1AdcMax2/1 -> Subtract1/1
  cmdTorqueMin/1 -> Subtract2/2
  Subtract2/1 -> Product/2
  cmdTorqueMax/1 -> Subtract2/1
  Subtract/1 -> Divide/1
  apps1AdcMin2/1 -> Add/1
  In1/1 -> Subtract/1
  In2/1 -> Product1/1
  Constant/1 -> Product1/2
  Product1/1 -> MATLAB Function/1(Speed)
  Divide/1 -> MATLAB Function/2(Apps)
  MATLAB Function/1(y) -> Product/1

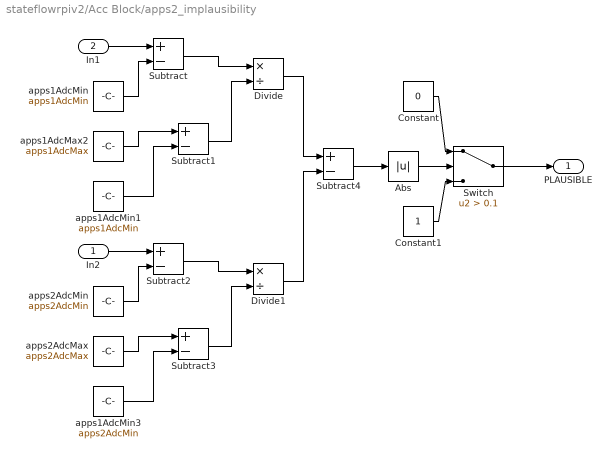
== system stateflowrpiv2/Acc Block/apps2_implausibility ==
  In2 : Inport
  In1 : Inport  Port=2
  Abs : Abs  SaturateOnIntegerOverflow=off
  Constant : Constant  Value=0
  Constant1 : Constant
  Divide : Product  Inputs=*/
  Divide1 : Product  Inputs=*/
  Subtract{,1..4} (5 alike) : Sum  Inputs=+-
  Switch : Switch  Criteria=u2 > Threshold  Threshold=0.1  SaturateOnIntegerOverflow=off  InputSameDT=off
  apps1AdcMax2 : Constant  Value=apps1AdcMax
  apps1AdcMin : Constant  Value=apps1AdcMin
  apps1AdcMin1 : Constant  Value=apps1AdcMin
  apps1AdcMin3 : Constant  Value=apps2AdcMin
  apps2AdcMax : Constant  Value=apps2AdcMax
  apps2AdcMin : Constant  Value=apps2AdcMin
  PLAUSIBLE : Outport
  wires:
  apps1AdcMin1/1 -> Subtract1/2
  apps1AdcMin/1 -> Subtract/2
  Subtract1/1 -> Divide/2
  apps1AdcMax2/1 -> Subtract1/1
  Subtract/1 -> Divide/1
  In1/1 -> Subtract/1
  apps1AdcMin3/1 -> Subtract3/2
  Subtract3/1 -> Divide1/2
  In2/1 -> Subtract2/1
  apps2AdcMax/1 -> Subtract3/1
  Subtract2/1 -> Divide1/1
  apps2AdcMin/1 -> Subtract2/2
  Subtract4/1 -> Abs/1
  Abs/1 -> Switch/2
  Divide/1 -> Subtract4/1
  Divide1/1 -> Subtract4/2
  Switch/1 -> PLAUSIBLE/1
  Constant/1 -> Switch/1
  Constant1/1 -> Switch/3

== system stateflowrpiv2/Inputs/If Action Subsystem ==
  In1 : Inport
  Action Port : ActionPort  ActionPortLabel=if(u1 == 0)
  TSON : Outport
  wires:
  In1/1 -> TSON/1

== system stateflowrpiv2/Inputs/If Action Subsystem1 ==
  In1 : Inport
  Action Port : ActionPort  ActionPortLabel=if(u1 == 0)
  TSON : Outport
  wires:
  In1/1 -> TSON/1

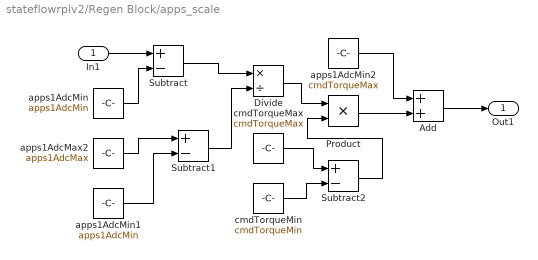
== system stateflowrpiv2/Regen Block/apps_scale ==
  In1 : Inport
  Add : Sum
  Divide : Product  Inputs=*/
  Product : Product
  Subtract : Sum  Inputs=+-
  Subtract1 : Sum  Inputs=+-
  Subtract2 : Sum  Inputs=+-
  apps1AdcMax2 : Constant  Value=apps1AdcMax
  apps1AdcMin : Constant  Value=apps1AdcMin
  apps1AdcMin1 : Constant  Value=apps1AdcMin
  apps1AdcMin2 : Constant  Value=cmdTorqueMax
  cmdTorqueMax : Constant  Value=cmdTorqueMax
  cmdTorqueMin : Constant  Value=cmdTorqueMin
  Out1 : Outport
  wires:
  Add/1 -> Out1/1
  Product/1 -> Add/2
  apps1AdcMin1/1 -> Subtract1/2
  apps1AdcMin/1 -> Subtract/2
  Subtract1/1 -> Divide/2
  Divide/1 -> Product/1
  apps1AdcMax2/1 -> Subtract1/1
  cmdTorqueMin/1 -> Subtract2/2
  Subtract2/1 -> Product/2
  cmdTorqueMax/1 -> Subtract2/1
  Subtract/1 -> Divide/1
  apps1AdcMin2/1 -> Add/1
  In1/1 -> Subtract/1

== matlab function stateflowrpiv2/Acc Block/MATLAB Function ==
  data: u input; y output; acc input; skid input; endu input
function y = fcn(u, acc, skid, endu)
if u==0
    y=acc;
elseif u==1
    y=endu;
elseif u==2
    y=skid;
end 

end

== matlab function stateflowrpiv2/Acc Block/apps1_scaleSkidpad/MATLAB Function ==
  data: Speed input; y output; Apps input
function y= fcn(Speed, Apps)
persistent prev_state;  % Retains value between function calls
    if isempty(prev_state)
        prev_state = 0;  % Initialize only once
    end
if(Speed>10.14) || (Speed<10.12)
    y = Apps;
    prev_state = Apps;
else
    if(Apps >= prev_state-0.1) && (Apps<=prev_state+0.3)
        y = prev_state;
    else
        y = Apps;
        prev_state = Apps;
    end
end

== stateflow chart stateflowrpiv2/STATEMACHINE ==
  state SDCTEST
    entry:
    ECUSDC=1;
  state TSON
    TSFlag=1;
    STFlag=0;
    ECUSDC=1;
    MCPOW=1;
  state TSOFF
    entry:
    TSFlag=0;
    STFlag=0;
    ECUSDC=0;
    MCPOW=0;
  state STRT
    on after(5,sec):
    Buzzer=0;
    state ACCEL
      EventFlag=0;
    state ENDURANCE
      EventFlag=1;
    state SKIDPAD
      EventFlag=2;
    STRT -> ACCEL [order 1] : [EVENT==0]
    ACCEL -> STRT
    SKIDPAD -> STRT
    ENDURANCE -> STRT
    (default) -> ENDURANCE
    STRT -> ENDURANCE [order 2] : [EVENT==1]
    STRT -> SKIDPAD [order 3] : [EVENT==2]
  TSON -> TSOFF [order 1] : [FINALSDC==0]
  (default) -> TSOFF
  TSOFF -> SDCTEST : [TSON==1]
  SDCTEST -> TSON [order 1] : [FINALSDC==1]
  SDCTEST -> TSOFF [order 2] : [FINALSDC==0]
  TSON -> STRT [order 2] : [STARTER==1 & FINALSDC==1]
      | {STFlag=1;
      | Buzzer=1;}
  STRT -> TSOFF [order 1] : [FINALSDC==0]
  data: FINALSDC input; TSON input; STARTER input; Buzzer output; TSFlag output; MCPOW output; STFlag output; ECUSDC output; EventFlag output; EVENT input
